simulink library "VelocityDALQR_lib"  (R2020b)
settings: Solver=VariableStepAuto  StartTime=0.0  StopTime=10.0  RelTol=1e-3
settings Model: Creator=Christian  LastModifiedBy=Christian

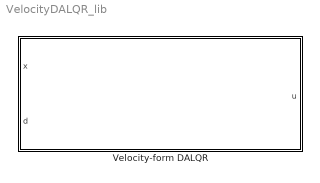
== system VelocityDALQR_lib ==
  Velocity-form DALQR : Subsystem  mask{K=[], B_disturbance=0, B=0}
      mask prompts: K "Gain Matrix"; B_disturbance "Disturbance Matrix"; B "Input Matrix"

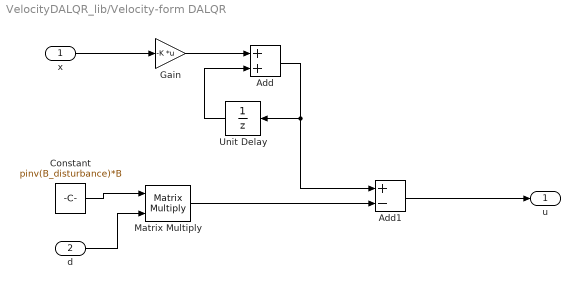
== system VelocityDALQR_lib/Velocity-form DALQR ==
  x : Inport
  d : Inport  Port=2
  Add : Sum
  Add1 : Sum  Inputs=+-
  Constant : Constant  Value=pinv(B_disturbance)*B  VectorParams1D=off
  Gain : Gain  Gain=-K  Multiplication=Matrix(K*u)
  Matrix Multiply : Product  Multiplication=Matrix(*)
  Unit Delay : UnitDelay  SampleTime=-1  HasFrameUpgradeWarning=on
  u : Outport
  wires:
  Add1/1 -> u/1
  Matrix Multiply/1 -> Add1/2
  Add/1 -> Add1/1, Unit Delay/1
  Gain/1 -> Add/1
  Unit Delay/1 -> Add/2
  x/1 -> Gain/1
  Constant/1 -> Matrix Multiply/1
  d/1 -> Matrix Multiply/2
